simulink library "Lib_Vol_pipeCd_TMATS_org"  (Simulink 10.0)
settings: Solver=ode45  StartTime=0.0  StopTime=10.0  RelTol=1e-3  EnableMultiTasking=on
undefined symbols (not defined in the file): Fluid
libraries: Lib_Vol_PropLookup_TMATS x3, simulink x1
Description:
  | Thomas Modules
settings Model: Creator=jwchapm2  LastModifiedBy=bhisma

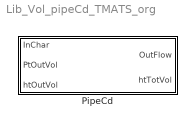
== system Lib_Vol_pipeCd_TMATS_org ==
  PipeCd : Subsystem  TreatAsAtomicUnit=on  mask(T-MATS: Duct Library Block){Cd_M=1, A_M=1, htVec_M=Fluid.Vec.ht, PtVec_M=Fluid.Vec.Pt, TtArray_M=Fluid.Array.Tt, rhoArray_M=Fluid.Array.rho}
      mask prompts: Cd_M "Cd_M - constant"; A_M "A_M - Area [in2]"; htVec_M "htVec_M - Temperature Vector"; PtVec_M "PtVec_M - Pressure Vector"; TtArray_M "TtArray_M - Total Temperature Array f(ht,Pt)"; rhoArray_M "rhoArray_M - density f(ht,Pt)"
      mask help: This block simulates the performance of a duct using basic fluid dynamic equations and properties.
      mask Help: web(which('Vol_TMATS_pipeCd.html'),'-helpbrowser')

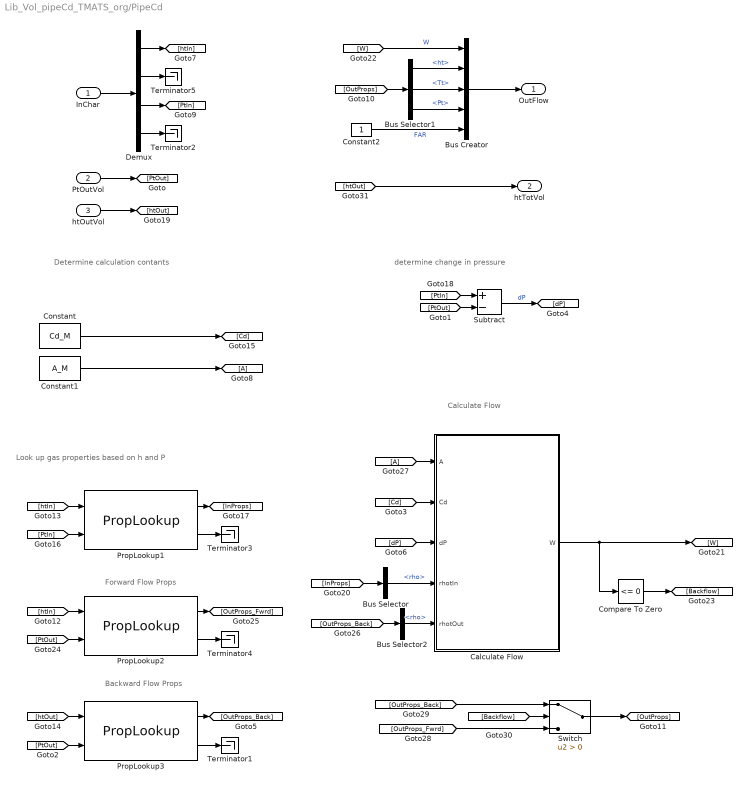
== system Lib_Vol_pipeCd_TMATS_org/PipeCd ==
  note: Look up gas properties based on h and P
  note: Calculate Flow
  note: Determine calculation contants
  note: determine change in pressure
  note: Backward Flow Props
  note: Forward Flow Props
  InChar : Inport
  PtOutVol : Inport  Port=2
  htOutVol : Inport  Port=3
  Bus Creator : BusCreator  Inputs=5
  Bus Selector : BusSelector  OutputSignals=rho
  Bus Selector1 : BusSelector  OutputSignals=ht,Tt,Pt
  Bus Selector2 : BusSelector  OutputSignals=rho
  Calculate Flow : MATLAB Function  TreatAsAtomicUnit=on
  Compare To Zero : simulink/Logic and Bit Operations/Compare To Zero  relop=<=  OutDataTypeStr=boolean
  Constant : Constant  Value=Cd_M
  Constant1 : Constant  Value=A_M
  Constant2 : Constant
  Demux : Demux
  PropLookup1 : Lib_Vol_PropLookup_TMATS/PropLookup  case_M='ht'  propg_M=0  htg_M=0  htVec_M=htVec_M  PtVec_M=PtVec_M  TtVec_M=[-10000 10000]  sVec_M=[-10000 10000]  htArray_M=ones(2, length(PtVec_M))'  rhoArray_M=rhoArray_M  uArray_M=ones(length(htVec_M), length(PtVec_M))'  sArray_M=ones(length(htVec_M), length(PtVec_M))'  muArray_M=ones(length(htVec_M), length(PtVec_M))'  ThArray_M=TtArray_M  CvArray_M=ones(length(htVec_M), length(PtVec_M))'  CpArray_M=ones(length(htVec_M), length(PtVec_M))'  kArray_M=ones(length(htVec_M), length(PtVec_M))'  TsArray_M=ones(2, length(PtVec_M))'  hsArray_M=ones(2, length(PtVec_M))'  Rval_M=0
  PropLookup2 : Lib_Vol_PropLookup_TMATS/PropLookup  case_M='ht'  propg_M=0  htg_M=0  htVec_M=htVec_M  PtVec_M=PtVec_M  TtVec_M=[-10000 10000]  sVec_M=[-10000 10000]  htArray_M=ones(2, length(PtVec_M))'  rhoArray_M=rhoArray_M  uArray_M=ones(length(htVec_M), length(PtVec_M))'  sArray_M=ones(length(htVec_M), length(PtVec_M))'  muArray_M=ones(length(htVec_M), length(PtVec_M))'  ThArray_M=TtArray_M  CvArray_M=ones(length(htVec_M), length(PtVec_M))'  CpArray_M=ones(length(htVec_M), length(PtVec_M))'  kArray_M=ones(length(htVec_M), length(PtVec_M))'  TsArray_M=ones(2, length(PtVec_M))'  hsArray_M=ones(2, length(PtVec_M))'  Rval_M=0
  PropLookup3 : Lib_Vol_PropLookup_TMATS/PropLookup  case_M='ht'  propg_M=0  htg_M=0  htVec_M=htVec_M  PtVec_M=PtVec_M  TtVec_M=[-10000 10000]  sVec_M=[-10000 10000]  htArray_M=ones(2, length(PtVec_M))'  rhoArray_M=rhoArray_M  uArray_M=ones(length(htVec_M), length(PtVec_M))'  sArray_M=ones(length(htVec_M), length(PtVec_M))'  muArray_M=ones(length(htVec_M), length(PtVec_M))'  ThArray_M=TtArray_M  CvArray_M=ones(length(htVec_M), length(PtVec_M))'  CpArray_M=ones(length(htVec_M), length(PtVec_M))'  kArray_M=ones(length(htVec_M), length(PtVec_M))'  TsArray_M=ones(2, length(PtVec_M))'  hsArray_M=ones(2, length(PtVec_M))'  Rval_M=0
  Subtract : Sum  Inputs=+-
  Switch : Switch  Criteria=u2 > Threshold
  Terminator{1..5} (5 alike) : Terminator
  OutFlow : Outport  PortDimensions=5
  htTotVol : Outport  Port=2  PortDimensions=1
  wires:
  Subtract/1 -> [dP]  "dP"
  PropLookup3/1 -> [OutProps_Back]
  PropLookup3/2 -> Terminator1/1
  PtOutVol/1 -> [PtOut]
  [PtOut] -> Subtract/2
  [PtOut] -> PropLookup3/2
  [htOut] -> PropLookup3/1
  Constant/1 -> [Cd]
  [PtIn] -> Subtract/1
  htOutVol/1 -> [htOut]
  [Cd] -> Calculate Flow/2(Cd)
  [dP] -> Calculate Flow/3(dP)
  InChar/1 -> Demux/1
  Demux/1 -> [htIn]
  Demux/4 -> Terminator2/1
  Demux/3 -> [PtIn]
  Demux/2 -> Terminator5/1
  PropLookup1/1 -> [InProps]
  PropLookup1/2 -> Terminator3/1
  [PtIn] -> PropLookup1/2
  [htIn] -> PropLookup1/1
  [InProps] -> Bus Selector/1
  Bus Selector/1 -> Calculate Flow/4(rhotIn)  "<rho>"
  [W] -> Bus Creator/1  "W"
  [OutProps] -> Bus Selector1/1
  Bus Selector1/1 -> Bus Creator/2  "<ht>"
  Bus Selector1/2 -> Bus Creator/3  "<Tt>"
  Bus Selector1/3 -> Bus Creator/4  "<Pt>"
  Constant2/1 -> Bus Creator/5  "FAR"
  Bus Creator/1 -> OutFlow/1
  [htOut] -> htTotVol/1
  Calculate Flow/1(W) -> Compare To Zero/1, [W]
  Compare To Zero/1 -> [Backflow]
  Switch/1 -> [OutProps]
  [OutProps_Back] -> Switch/1
  [OutProps_Fwrd] -> Switch/3
  [Backflow] -> Switch/2
  PropLookup2/1 -> [OutProps_Fwrd]
  PropLookup2/2 -> Terminator4/1
  [PtOut] -> PropLookup2/2
  [htIn] -> PropLookup2/1
  Bus Selector2/1 -> Calculate Flow/5(rhotOut)  "<rho>"
  [OutProps_Back] -> Bus Selector2/1
  Constant1/1 -> [A]
  [A] -> Calculate Flow/1(A)

== matlab function PipeCd/Calculate Flow ==
  data: A input double; Cd input double; W output double; dP input double; rhotIn input double; rhotOut input double
function W = fcn(A,Cd,dP,rhotIn, rhotOut)
%#codegen

g = 32.174049;
if dP > 0
    W = Cd*A*sqrt(2*g*dP *( rhotIn/12/12/12 ));  %LBM/SEC
else
    W = -Cd*A*sqrt(2*g*-dP *( rhotOut/12/12/12 ));  %LBM/SEC 
end
